simulink model "pd_control_v3"  (R2022b)
settings: Solver=VariableStepAuto  StartTime=0.0  StopTime=5  RelTol=1e-3
values from neighbouring files (symbols this model uses):
  m = 6    [coordinator_v2.m]
  N = 10    [coordinator_v2.m]
undefined symbols (not defined in the file or in its folder): X, Y, Z
libraries: sm_lib x191, nesl_utility x71
(part 5 of 5)

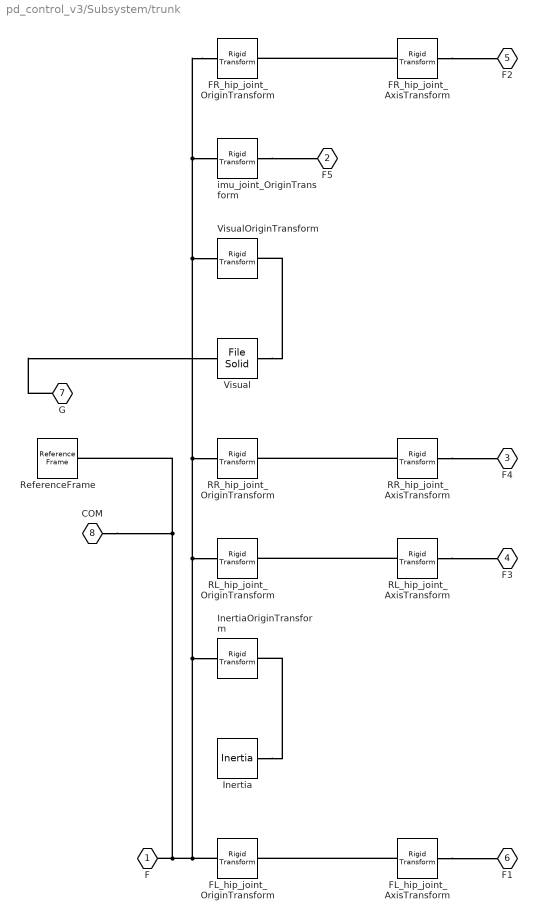
== system pd_control_v3/Subsystem/trunk ==
  FL_hip_joint_AxisTransform : sm_lib/Frames and Transforms/Rigid Transform  TranslationMethod=Cartesian  TranslationStandardOffset=0  TranslationLengthUnit=m  TranslationStandardAxis=+Z  TranslationCartesianOffset=[0, 0, 0]  TranslationROffset=0  TranslationROffsetUnits=m  TranslationZOffset=0  TranslationZOffsetUnits=m  TranslationThetaOffset=0  TranslationThetaOffsetUnits=deg  RotationMethod=ArbitraryAxis  RotationAngleUnits=rad  RotationStandardAxis=+Z  RotationAngle=1.570796326794897  RotationArbitraryAxis=[-0, 1, 0]  FollAlignAxisA=+X  BaseAlignAxisA=+Y  FollAlignAxisB=+Y  BaseAlignAxisB=+Z  RotationSequenceAxes=FollowerAxes  RotationSequence=XYX  RotationSequenceAngles=[0 0 0]  RotationSequenceAnglesUnits=deg  RotationMatrix=[1 0 0; 0 1 0; 0 0 1]  Quaternion=[1 0 0 0]
  FL_hip_joint_OriginTransform : sm_lib/Frames and Transforms/Rigid Transform  TranslationMethod=Cartesian  TranslationStandardOffset=0  TranslationLengthUnit=m  TranslationStandardAxis=+Z  TranslationCartesianOffset=[0.1805, 0.047, 0]  TranslationROffset=0  TranslationROffsetUnits=m  TranslationZOffset=0  TranslationZOffsetUnits=m  TranslationThetaOffset=0  TranslationThetaOffsetUnits=deg  RotationMethod=RotationSequence  RotationAngleUnits=deg  RotationStandardAxis=+Z  RotationAngle=0.0  RotationArbitraryAxis=[0 0 1]  FollAlignAxisA=+X  BaseAlignAxisA=+Y  FollAlignAxisB=+Y  BaseAlignAxisB=+Z  RotationSequenceAxes=BaseAxes  RotationSequence=XYZ  RotationSequenceAngles=[0, 0, 0]  RotationSequenceAnglesUnits=rad  RotationMatrix=[1 0 0; 0 1 0; 0 0 1]  Quaternion=[1 0 0 0]
  FR_hip_joint_AxisTransform : sm_lib/Frames and Transforms/Rigid Transform  TranslationMethod=Cartesian  TranslationStandardOffset=0  TranslationLengthUnit=m  TranslationStandardAxis=+Z  TranslationCartesianOffset=[0, 0, 0]  TranslationROffset=0  TranslationROffsetUnits=m  TranslationZOffset=0  TranslationZOffsetUnits=m  TranslationThetaOffset=0  TranslationThetaOffsetUnits=deg  RotationMethod=ArbitraryAxis  RotationAngleUnits=rad  RotationStandardAxis=+Z  RotationAngle=1.570796326794897  RotationArbitraryAxis=[-0, 1, 0]  FollAlignAxisA=+X  BaseAlignAxisA=+Y  FollAlignAxisB=+Y  BaseAlignAxisB=+Z  RotationSequenceAxes=FollowerAxes  RotationSequence=XYX  RotationSequenceAngles=[0 0 0]  RotationSequenceAnglesUnits=deg  RotationMatrix=[1 0 0; 0 1 0; 0 0 1]  Quaternion=[1 0 0 0]
  FR_hip_joint_OriginTransform : sm_lib/Frames and Transforms/Rigid Transform  TranslationMethod=Cartesian  TranslationStandardOffset=0  TranslationLengthUnit=m  TranslationStandardAxis=+Z  TranslationCartesianOffset=[0.1805, -0.047, 0]  TranslationROffset=0  TranslationROffsetUnits=m  TranslationZOffset=0  TranslationZOffsetUnits=m  TranslationThetaOffset=0  TranslationThetaOffsetUnits=deg  RotationMethod=RotationSequence  RotationAngleUnits=deg  RotationStandardAxis=+Z  RotationAngle=0.0  RotationArbitraryAxis=[0 0 1]  FollAlignAxisA=+X  BaseAlignAxisA=+Y  FollAlignAxisB=+Y  BaseAlignAxisB=+Z  RotationSequenceAxes=BaseAxes  RotationSequence=XYZ  RotationSequenceAngles=[0, 0, 0]  RotationSequenceAnglesUnits=rad  RotationMatrix=[1 0 0; 0 1 0; 0 0 1]  Quaternion=[1 0 0 0]
  Inertia : sm_lib/Body Elements/Inertia  InertiaType=Custom  Mass=6  MassUnits=kg  CenterOfMass=[0, 0, 0]  CenterOfMassUnits=m  MomentsOfInertia=[0.0158533, 0.0377999, 0.0456542]  MomentsOfInertiaUnits=kg*m^2  ProductsOfInertia=[-2.75e-05, -6.109999999999999e-05, -3.66e-05]  ProductsOfInertiaUnits=kg*m^2  GraphicType=None  MarkerShape=Inertia  MarkerSize=20  GraphicVisPropType=SimpleVisualProperties  GraphicDiffuseColor=[0.5 0.5 0.5]  GraphicSpecularColor=[0.5 0.5 0.5 1.0]  GraphicAmbientColor=[0.15 0.15 0.15 1.0]  GraphicEmissiveColor=[0.0 0.0 0.0 1.0]  GraphicShininess=75  GraphicOpacity=1.0
  InertiaOriginTransform : sm_lib/Frames and Transforms/Rigid Transform  TranslationMethod=Cartesian  TranslationStandardOffset=0  TranslationLengthUnit=m  TranslationStandardAxis=+Z  TranslationCartesianOffset=[0, 0.0041, -0.0005]  TranslationROffset=0  TranslationROffsetUnits=m  TranslationZOffset=0  TranslationZOffsetUnits=m  TranslationThetaOffset=0  TranslationThetaOffsetUnits=deg  RotationMethod=RotationSequence  RotationAngleUnits=deg  RotationStandardAxis=+Z  RotationAngle=0.0  RotationArbitraryAxis=[0 0 1]  FollAlignAxisA=+X  BaseAlignAxisA=+Y  FollAlignAxisB=+Y  BaseAlignAxisB=+Z  RotationSequenceAxes=BaseAxes  RotationSequence=XYZ  RotationSequenceAngles=[0, 0, 0]  RotationSequenceAnglesUnits=rad  RotationMatrix=[1 0 0; 0 1 0; 0 0 1]  Quaternion=[1 0 0 0]
  RL_hip_joint_AxisTransform : sm_lib/Frames and Transforms/Rigid Transform  TranslationMethod=Cartesian  TranslationStandardOffset=0  TranslationLengthUnit=m  TranslationStandardAxis=+Z  TranslationCartesianOffset=[0, 0, 0]  TranslationROffset=0  TranslationROffsetUnits=m  TranslationZOffset=0  TranslationZOffsetUnits=m  TranslationThetaOffset=0  TranslationThetaOffsetUnits=deg  RotationMethod=ArbitraryAxis  RotationAngleUnits=rad  RotationStandardAxis=+Z  RotationAngle=1.570796326794897  RotationArbitraryAxis=[-0, 1, 0]  FollAlignAxisA=+X  BaseAlignAxisA=+Y  FollAlignAxisB=+Y  BaseAlignAxisB=+Z  RotationSequenceAxes=FollowerAxes  RotationSequence=XYX  RotationSequenceAngles=[0 0 0]  RotationSequenceAnglesUnits=deg  RotationMatrix=[1 0 0; 0 1 0; 0 0 1]  Quaternion=[1 0 0 0]
  RL_hip_joint_OriginTransform : sm_lib/Frames and Transforms/Rigid Transform  TranslationMethod=Cartesian  TranslationStandardOffset=0  TranslationLengthUnit=m  TranslationStandardAxis=+Z  TranslationCartesianOffset=[-0.1805, 0.047, 0]  TranslationROffset=0  TranslationROffsetUnits=m  TranslationZOffset=0  TranslationZOffsetUnits=m  TranslationThetaOffset=0  TranslationThetaOffsetUnits=deg  RotationMethod=RotationSequence  RotationAngleUnits=deg  RotationStandardAxis=+Z  RotationAngle=0.0  RotationArbitraryAxis=[0 0 1]  FollAlignAxisA=+X  BaseAlignAxisA=+Y  FollAlignAxisB=+Y  BaseAlignAxisB=+Z  RotationSequenceAxes=BaseAxes  RotationSequence=XYZ  RotationSequenceAngles=[0, 0, 0]  RotationSequenceAnglesUnits=rad  RotationMatrix=[1 0 0; 0 1 0; 0 0 1]  Quaternion=[1 0 0 0]
  RR_hip_joint_AxisTransform : sm_lib/Frames and Transforms/Rigid Transform  TranslationMethod=Cartesian  TranslationStandardOffset=0  TranslationLengthUnit=m  TranslationStandardAxis=+Z  TranslationCartesianOffset=[0, 0, 0]  TranslationROffset=0  TranslationROffsetUnits=m  TranslationZOffset=0  TranslationZOffsetUnits=m  TranslationThetaOffset=0  TranslationThetaOffsetUnits=deg  RotationMethod=ArbitraryAxis  RotationAngleUnits=rad  RotationStandardAxis=+Z  RotationAngle=1.570796326794897  RotationArbitraryAxis=[-0, 1, 0]  FollAlignAxisA=+X  BaseAlignAxisA=+Y  FollAlignAxisB=+Y  BaseAlignAxisB=+Z  RotationSequenceAxes=FollowerAxes  RotationSequence=XYX  RotationSequenceAngles=[0 0 0]  RotationSequenceAnglesUnits=deg  RotationMatrix=[1 0 0; 0 1 0; 0 0 1]  Quaternion=[1 0 0 0]
  RR_hip_joint_OriginTransform : sm_lib/Frames and Transforms/Rigid Transform  TranslationMethod=Cartesian  TranslationStandardOffset=0  TranslationLengthUnit=m  TranslationStandardAxis=+Z  TranslationCartesianOffset=[-0.1805, -0.047, 0]  TranslationROffset=0  TranslationROffsetUnits=m  TranslationZOffset=0  TranslationZOffsetUnits=m  TranslationThetaOffset=0  TranslationThetaOffsetUnits=deg  RotationMethod=RotationSequence  RotationAngleUnits=deg  RotationStandardAxis=+Z  RotationAngle=0.0  RotationArbitraryAxis=[0 0 1]  FollAlignAxisA=+X  BaseAlignAxisA=+Y  FollAlignAxisB=+Y  BaseAlignAxisB=+Z  RotationSequenceAxes=BaseAxes  RotationSequence=XYZ  RotationSequenceAngles=[0, 0, 0]  RotationSequenceAnglesUnits=rad  RotationMatrix=[1 0 0; 0 1 0; 0 0 1]  Quaternion=[1 0 0 0]
  ReferenceFrame : sm_lib/Frames and Transforms/Reference Frame
  Visual : sm_lib/Body Elements/File Solid  ExtGeomFileName=a1_description\meshes\trunk.stl  UnitType=Custom  ExtGeomFileUnits=m  StepReaderType=HEX  ExportConvexHullGeometry=on  InertiaType=Custom  Mass=0  MassUnits=kg  CenterOfMass=[0, 0, 0]  CenterOfMassUnits=m  MomentsOfInertia=[0, 0, 0]  MomentsOfInertiaUnits=kg*m^2  ProductsOfInertia=[0, 0, 0]  ProductsOfInertiaUnits=kg*m^2  BasedOnType=DensityFromFile  Density=1000  DensityUnits=kg/m^3  DoExposeReferenceFrame=on  SerializedFrames=<Frames/>  GraphicType=FromGeometry  MarkerShape=Sphere  MarkerSize=10  GraphicVisPropType=SimpleVisualProperties  GraphicDiffuseColor=[1, 0.423529411765, 0.0392156862745]  GraphicSpecularColor=[0.5 0.5 0.5 1.0]  GraphicAmbientColor=[0.15 0.15 0.15 1.0]  GraphicEmissiveColor=[0.0 0.0 0.0 1.0]  GraphicShininess=75  GraphicOpacity=1
  VisualOriginTransform : sm_lib/Frames and Transforms/Rigid Transform  TranslationMethod=Cartesian  TranslationStandardOffset=0  TranslationLengthUnit=m  TranslationStandardAxis=+Z  TranslationCartesianOffset=[0, 0, 0]  TranslationROffset=0  TranslationROffsetUnits=m  TranslationZOffset=0  TranslationZOffsetUnits=m  TranslationThetaOffset=0  TranslationThetaOffsetUnits=deg  RotationMethod=RotationSequence  RotationAngleUnits=deg  RotationStandardAxis=+Z  RotationAngle=0.0  RotationArbitraryAxis=[0 0 1]  FollAlignAxisA=+X  BaseAlignAxisA=+Y  FollAlignAxisB=+Y  BaseAlignAxisB=+Z  RotationSequenceAxes=BaseAxes  RotationSequence=XYZ  RotationSequenceAngles=[0, 0, 0]  RotationSequenceAnglesUnits=rad  RotationMatrix=[1 0 0; 0 1 0; 0 0 1]  Quaternion=[1 0 0 0]
  imu_joint_OriginTransform : sm_lib/Frames and Transforms/Rigid Transform  TranslationMethod=Cartesian  TranslationStandardOffset=0  TranslationLengthUnit=m  TranslationStandardAxis=+Z  TranslationCartesianOffset=[0, 0, 0]  TranslationROffset=0  TranslationROffsetUnits=m  TranslationZOffset=0  TranslationZOffsetUnits=m  TranslationThetaOffset=0  TranslationThetaOffsetUnits=deg  RotationMethod=RotationSequence  RotationAngleUnits=deg  RotationStandardAxis=+Z  RotationAngle=0.0  RotationArbitraryAxis=[0 0 1]  FollAlignAxisA=+X  BaseAlignAxisA=+Y  FollAlignAxisB=+Y  BaseAlignAxisB=+Z  RotationSequenceAxes=BaseAxes  RotationSequence=XYZ  RotationSequenceAngles=[0, 0, 0]  RotationSequenceAnglesUnits=rad  RotationMatrix=[1 0 0; 0 1 0; 0 0 1]  Quaternion=[1 0 0 0]
  F : PMIOPort  Side=Left
  F5 : PMIOPort  Port=2  Side=Right
  F4 : PMIOPort  Port=3  Side=Right
  F3 : PMIOPort  Port=4  Side=Right
  F2 : PMIOPort  Port=5  Side=Right
  F1 : PMIOPort  Port=6  Side=Right
  G : PMIOPort  Port=7  Side=Right
  COM : PMIOPort  Port=8  Side=Right
  connections:
  FL_hip_joint_AxisTransform/RConn1 -- F1/RConn1
  FL_hip_joint_AxisTransform/LConn1 -- FL_hip_joint_OriginTransform/RConn1
  FR_hip_joint_AxisTransform/RConn1 -- F2/RConn1
  FR_hip_joint_AxisTransform/LConn1 -- FR_hip_joint_OriginTransform/RConn1
  Inertia/RConn1 -- InertiaOriginTransform/RConn1
  RL_hip_joint_AxisTransform/RConn1 -- F3/RConn1
  RL_hip_joint_AxisTransform/LConn1 -- RL_hip_joint_OriginTransform/RConn1
  RR_hip_joint_AxisTransform/RConn1 -- F4/RConn1
  RR_hip_joint_AxisTransform/LConn1 -- RR_hip_joint_OriginTransform/RConn1
  FR_hip_joint_OriginTransform/LConn1 -- FL_hip_joint_OriginTransform/LConn1 -- COM/RConn1 -- ReferenceFrame/RConn1 -- F/RConn1 -- InertiaOriginTransform/LConn1 -- RL_hip_joint_OriginTransform/LConn1 -- RR_hip_joint_OriginTransform/LConn1 -- VisualOriginTransform/LConn1 -- imu_joint_OriginTransform/LConn1
  Visual/RConn1 -- VisualOriginTransform/RConn1
  imu_joint_OriginTransform/RConn1 -- F5/RConn1
  G/RConn1 -- Visual/LConn1

== matlab function pd_control_v3/MPC Controller ==
  data: q input; y output; t input; r input; dt input; N input; sd input
% Input:
% System state: s, (12, 1)
% time: t
% mode: mode, indicating which foot on ground
% foot positions: r = [r_front_left; r_front_right; r_rear_left;
% r_rear_right]
% Inertial of body: Ib
% body mass: m
% time step: dt
% MPC horizon length: N
% Desired system state: sd
% Output:
% Foot force: y = [F_front_left; F_front_right; F_rear_left;
% F_rear_right]: 
% q: [x; y; z; roll; pitch; yaw; dx; dy; dz; w]
% sd: [xd; yd; zd; roll_d; pitch_d; yaw_d; dx_d; dy_d; dz_d; w_d]
% r: foot positions in world frame
%% Controller functions
% q: [x; y; z; roll; pitch; yaw; dx; dy; dz; w]
% sd: [xd; yd; zd; roll_d; pitch_d; yaw_d; dx_d; dy_d; dz_d; w_d]
% r: foot positions in world frame
function y = MPC_cntr_wrapper(q, t, r, dt, N, sd)
    Ib = [0.0168, 0, 0;
        0, 0.0565, 0;
        0, 0, 0.064];
    m = 6;
    mode_list = [];
    iteration = floor(mod(t/dt,N));
    disp(t);
    disp(iteration);
    
    for i = 0:N-1
        iter = mod((i +1 + iteration), N);
        if iter <= N / 2
            mode_list = [mode_list; 1];
        else
            mode_list = [mode_list; 2];
        end
    end
    disp(transpose(mode_list));
    y = MPC_controller(q, t, mode_list, r, Ib, m, dt, N, sd);
end

function y = MPC_controller(q, t, mode_list, r, Ib, m, dt, N, sd)
    p = q(1:3);
    eul = q(4:6);
    dp = q(7:9);
    wb = q(10:12);
    
    r1 = r(1:3) - p;
    r2 = r(4:6) - p;
    r3 = r(7:9) - p;
    r4 = r(10:12) - p;
    xd = sd;
    Q_mpc = diag([40,50,60,10,10,10,4,4,4,1,1,1]);
    R_mpc = 0.00001 * eye(12);

    state_num = 13;
    controller_num = 12;
    
    q0 = q;
    
    [Act, Bct]=linearize(q, [r1; r2; r3; r4], Ib, m, sd);
    
    Q_mpc = blkdiag(Q_mpc,0);
    xd = [xd;9.8];
    
    QCell = repmat({Q_mpc}, 1, N);
    RCell = repmat({R_mpc}, 1, N);
    H = blkdiag(QCell{:}, RCell{:});
    f_blk = -Q_mpc*xd;
    f = [repmat(f_blk, N, 1);zeros(N*controller_num,1)];
    
    [Aeq, Beq] = get_equality_constraint([q0; 9.81], Act, Bct, dt, N);

    Aineq = [];
    Bineq = [];

    for i=1:N
        mode = mode_list(i);
        if mode == 0
            [Ain, Bin] = MPC_all_foot();
            Aineq = blkdiag(Aineq, Ain);
            Bineq = [Bineq; Bin];
        elseif mode == 1
            [Ain, Bin] = MPC_fl_rr_foot();
            Aineq = blkdiag(Aineq, Ain);
            Bineq = [Bineq; Bin];
        elseif mode == 2
            [Ain, Bin] = MPC_fr_rl_foot();
            Aineq = blkdiag(Aineq, Ain);
            Bineq = [Bineq; Bin];
        elseif mode == 3
            [Ain, Bin] = MPC_f_foot();
            Aineq = blkdiag(Aineq, Ain);
            Bineq = [Bineq; Bin];
        elseif mode == 4
            [Ain, Bin] = MPC_r_foot();
            Aineq = blkdiag(Aineq, Ain);
            Bineq = [Bineq; Bin];
        end
    end

    A_sz = size(Aineq);
    Aineq = [zeros(A_sz(1), state_num * N), Aineq];
%     disp(Aineq);

    options = optimoptions('quadprog','Display','off');
    X_star = quadprog(H,f,Aineq,Bineq,Aeq,Beq,[],[],[],options);

    y = X_star(N*state_num+1:N*state_num+controller_num);
end

% mode = 0, Four foot on ground
function [Ain, Bin] = MPC_all_foot()
    [A, B]=singleIneq();
    A_sz = size(A);
    Ain = A;
    Bin = B;
end

% mode = 1, front left and rear right on ground
function [Ain, Bin] = MPC_fl_rr_foot()
    [A, B]=singleIneq(); % F = [F1; F2; F3; F4], AF < B
    B(1 * 6 + 1) = 0;
    B(1 * 6 + 2) = 0;
    B(2 * 6 + 1) = 0;
    B(2 * 6 + 2) = 0;

    Ain = A;
    Bin = B;
end

% mode = 2, front right and rear left on ground
function [Ain, Bin] = MPC_fr_rl_foot()
    [A, B]=singleIneq();
    B(0 * 6 + 1) = 0;
    B(0 * 6 + 2) = 0;
    B(3 * 6 + 1) = 0;
    B(3 * 6 + 2) = 0;
    
    Ain = A;
    Bin = B;
end

% mode = 3, both front on ground
function [Ain, Bin] = MPC_f_foot()
    [A, B]=singleIneq();
    B(0 * 6 + 1) = 0;
    B(0 * 6 + 2) = 0;
    B(1 * 6 + 1) = 0;
    B(1 * 6 + 2) = 0;
    
    Ain = A;
    Bin = B;
end

% mode = 4, both rear on ground
function [Ain, Bin] = MPC_r_foot()
    [A, B]=singleIneq();
    B(2 * 6 + 1) = 0;
    B(2 * 6 + 2) = 0;
    B(3 * 6 + 1) = 0;
    B(3 * 6 + 2) = 0;
    
    Ain = A;
    Bin = B;
end

%% utility functions
% Transformation matrix to transform euler angle velocity to angular
% velocity
function T=Trans_euler2angular(Theta)
    theta = Theta(2);
    Phi = Theta(3);
    T = [cos(Phi) * cos(theta), -sin(Phi), 0;
        sin(Phi) * cos(theta), cos(Phi), 0;
        -sin(theta), 0, 1];
end

% Skew matrix from vector
function S = vector2skewmat(a)
    S = [0 -a(3) a(2);
     a(3) 0 -a(1);
     -a(2) a(1) 0];
end

% Matrix A, B in linearization
% input:
% System state: s
% Foot positions: r = [r_front_left; r_front_right; r_rear_left;
% r_rear_right]
% Inertial in world frame: Iw
% body mass: m
function [Act, Bct]=linearize(s, r, Ib, m, sd)
    p = s(1:3);
    eul = s(4:6);
    dp = s(7:9);
    wb = s(10:12);
    r1 = r(1:3);
    r2 = r(4:6);
    r3 = r(7:9);
    r4 = r(10:12);
    
    R = eul2rotm([eul(3), eul(2), eul(1)]);
    yaw = eul(3);
    Rz_yaw = [cos(yaw) sin(yaw) 0;
             -sin(yaw) cos(yaw) 0;
             0 0 1];
    Act = [zeros(3) zeros(3) eye(3) zeros(3) zeros(3,1);
             zeros(3) zeros(3) zeros(3) Rz_yaw zeros(3,1);
             zeros(3) zeros(3) zeros(3) zeros(3) [0;0;-1];
             zeros(4,13)];
    Iw = R'*Ib*R;
    D = [m*eye(3) zeros(3);
         zeros(3) Iw];
    A = [eye(3), eye(3), eye(3), eye(3);
        vector2skewmat(r1),vector2skewmat(r2),vector2skewmat(r3),vector2skewmat(r4)];
    Bct = [zeros(6,12);
             D\A;
             zeros(1,12)];

end

function [Aeq, Beq]=get_equality_constraint(s, A, B, dt, N)
    A_bar = A * dt + eye(size(A));
    B_bar = B * dt;

    Aside = eye(size(A) * N);
    sz = size(A);
    for i=2:N
        row_start = (i-1) * sz(1) + 1;
        row_end = i * sz(1);
        col_start = (i-2) * sz(2) + 1;
        col_end = (i-1) * sz(2);
        Aside(row_start:row_end, col_start:col_end) = -A_bar;
    end

    BCell = repmat({-B_bar}, 1, N);
    Bside = blkdiag(BCell{:});
    Aeq = [Aside, Bside];
    Beq = zeros(N * 13, 1);
    Beq(1:13) = A_bar * s;
end

% F = [F1; F2; F3; F4] inequality constraint
function [A, B]=singleIneq()
    mu = 0.5;
    a = [0, 0, 1;
        0, 0, -1;
        1, 0, -mu;
        -1, 0, -mu;
        0, 1, -mu;
        0, -1, -mu];
    b = [500; -10; 0; 0; 0; 0];
    A = blkdiag(a, a, a, a);
    B = [b; b; b; b];
end

== matlab function pd_control_v3/MATLAB Function ==
  data: t input; q1 input; u1 output; q2 input; q3 input; q4 input; q5 input; q6 input; q7 input; q8 input; q9 input; q10 input; q11 input; q12 input; w1 input; w2 input; w3 input; w4 input; w5 input; w6 input; w7 input; w8 input; w9 input; w10 input; w11 input; w12 input; u2 output; u3 output; u4 output; u5 output; u6 output; u7 output; u8 output; u9 output; u10 output; u11 output; u12 output
function [u1,u2,u3,u4,u5,u6,u7,u8,u9,u10,u11,u12] = PD_constrol_standing(t,q1,q2,q3,q4,q5,q6,q7,q8,q9,q10,q11,q12,w1,w2,w3,w4,w5,w6,w7,w8,w9,w10,w11,w12)
    kp1 = 100;
    kv1 = 40;
    kp2 = 120;
    kv2 = 50;
    q1d = 0;
    q2d = 0;
    q3d = 0;
    q4d = 0;
    q5d = 0.5;
    q6d = 0.5;
    q7d = 0.5;
    q8d = 0.5;
    q9d = -1;
    q10d = -1;
    q11d = -1;
    q12d = -1;
    w1d = 0;
    w2d = 0;
    w3d = 0;
    w4d = 0;
    w5d = 0;
    w6d = 0;
    w7d = 0;
    w8d = 0;
    w9d = 0;
    w10d = 0;
    w11d = 0;
    w12d = 0;

    if t < 0.4
        u1 = 0;
        u2 = 0;
        u3 = 0;
        u4 = 0;
        u5 = 0;
        u6 = 0;
        u7 = 0;
        u8 = 0;
        u9 = 0;
        u10 = 0;
        u11 = 0;
        u12 = 0;
    
    else 
        u1 = kp1*(q1d-q1)+kv1*(w1d-w1);
        u2 = kp1*(q2d-q2)+kv1*(w2d-w2);
        u3 = kp2*(q3d-q3)+kv2*(w3d-w3);
        u4 = kp2*(q4d-q4)+kv2*(w4d-w4);
        u5 = kp1*(q5d-q5)+kv1*(w5d-w5);
        u6 = kp1*(q6d-q6)+kv1*(w6d-w6);
        u7 = kp2*(q7d-q7)+kv2*(w7d-w7);
        u8 = kp2*(q8d-q8)+kv2*(w8d-w8);
        u9 = kp1*(q9d-q9)+kv1*(w9d-w9);
        u10 = kp1*(q10d-q10)+kv1*(w10d-w10);
        u11 = kp2*(q11d-q11)+kv2*(w11d-w11);
        u12 = kp2*(q12d-q12)+kv2*(w12d-w12);

    end
end
